simulink model "create_obs"  (R2019a)
settings: Solver=FixedStepAuto  StartTime=0.0  StopTime=100  FixedStep=1/4000  RelTol=1e-3
settings Model: Creator=brandlju  LastModifiedBy=brandlju
settings OptimizationCC: LocalBlockOutputs=off
settings RTWCC: SystemTargetFile=TwinCAT.tlc  GenCodeOnly=on  MakeCommand=make_tct  TemplateMakefile=tct_msbuild.tmf  Description=TwinCAT Target  GenerateReport=on  TargetLang=C++
settings STFCustomTargetCC: TargetLangStandard=C++03 (ISO)  CompOptLevelCompliant=on  MATLABClassNameForMDSCustomization=Simulink.SoftwareTarget.TargetSpecificTriggerConfigurationBase  SystemTargetFile=TwinCAT.tlc

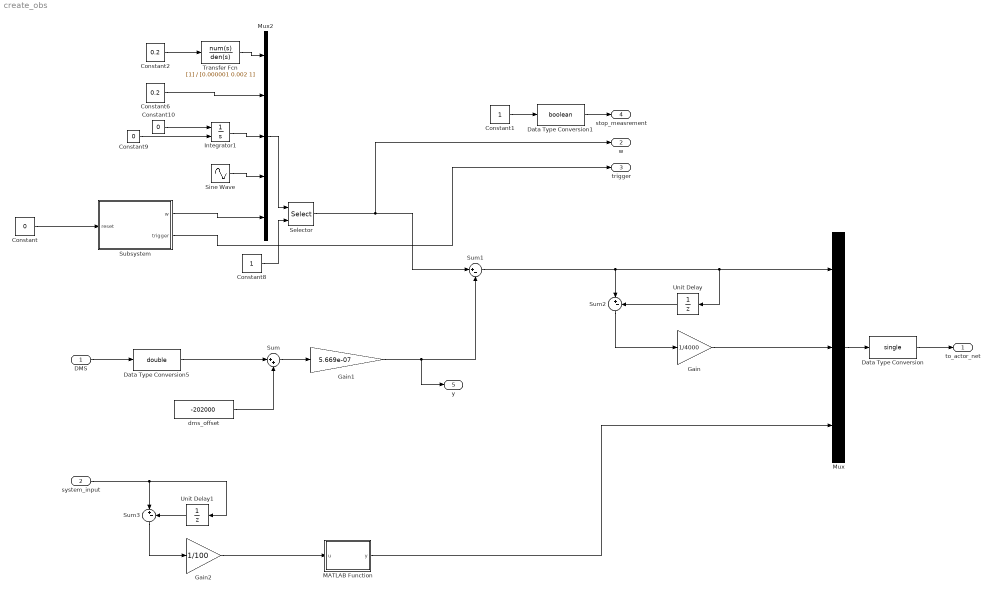
== system create_obs ==
  DMS : Inport  OutDataTypeStr=int32
  system_input : Inport  Port=2
  Constant : Constant  Value=0
  Constant1 : Constant
  Constant10 : Constant  Value=0
  Constant2 : Constant  Value=0.2
  Constant6 : Constant  Value=0.2
  Constant8 : Constant
  Constant9 : Constant  Value=0
  Data Type Conversion : DataTypeConversion  OutDataTypeStr=single
  Data Type Conversion1 : DataTypeConversion  OutDataTypeStr=boolean
  Data Type Conversion5 : DataTypeConversion  OutDataTypeStr=double
  Gain : Gain  Gain=1/4000
  Gain1 : Gain  Gain=5.669e-07
  Gain2 : Gain  Gain=1/100
  Integrator1 : Integrator  ExternalReset=either
  MATLAB Function : MATLAB Function  TreatAsAtomicUnit=on
  Mux : Mux  Inputs=3
  Mux2 : Mux  Inputs=5
  Selector : Selector  InputPortWidth=5  IndexOptions=Index vector (port)  Indices=[1 3]  OutputSizes=1
  Sine Wave : Sin  Amplitude=0.5  Bias=0.5  Frequency=0.1  SampleTime=0
  Subsystem : Subsystem
  Sum : Sum  Inputs=|++
  Sum1 : Sum  Inputs=|+-
  Sum2 : Sum  Inputs=|+-
  Sum3 : Sum  Inputs=|+-
  Transfer Fcn : TransferFcn  Denominator=[0.000001 0.002 1]
  Unit Delay : UnitDelay  SampleTime=-1  HasFrameUpgradeWarning=on
  Unit Delay1 : UnitDelay  SampleTime=-1  HasFrameUpgradeWarning=on
  "dms_offset " : Constant  Value=-202000
  to_actor_net : Outport  OutDataTypeStr=single
  w : Outport  Port=2
  trigger : Outport  Port=3
  stop_measrement : Outport  Port=4  OutDataTypeStr=boolean
  y : Outport  Port=5
  wires:
  "dms_offset "/1 -> Sum/2
  Data Type Conversion5/1 -> Sum/1
  Sum/1 -> Gain1/1
  DMS/1 -> Data Type Conversion5/1
  Gain1/1 -> y/1, Sum1/2
  Selector/1 -> w/1, Sum1/1
  Sum1/1 -> Sum2/1, Unit Delay/1, Mux/1
  Unit Delay/1 -> Sum2/2
  Gain/1 -> Mux/2
  Sum2/1 -> Gain/1
  Gain2/1 -> MATLAB Function/1(u)
  Sum3/1 -> Gain2/1
  system_input/1 -> Sum3/1, Unit Delay1/1
  Unit Delay1/1 -> Sum3/2
  MATLAB Function/1(y) -> Mux/3
  Mux/1 -> Data Type Conversion/1
  Data Type Conversion/1 -> to_actor_net/1
  Constant6/1 -> Mux2/2
  Sine Wave/1 -> Mux2/4
  Constant9/1 -> Integrator1/2
  Constant10/1 -> Integrator1/1
  Constant8/1 -> Selector/2
  Integrator1/1 -> Mux2/3
  Mux2/1 -> Selector/1
  Constant2/1 -> Transfer Fcn/1
  Transfer Fcn/1 -> Mux2/1
  Subsystem/1(w) -> Mux2/5
  Constant/1 -> Subsystem/1(reset)
  Data Type Conversion1/1 -> stop_measrement/1
  Constant1/1 -> Data Type Conversion1/1
  Subsystem/2(trigger) -> trigger/1

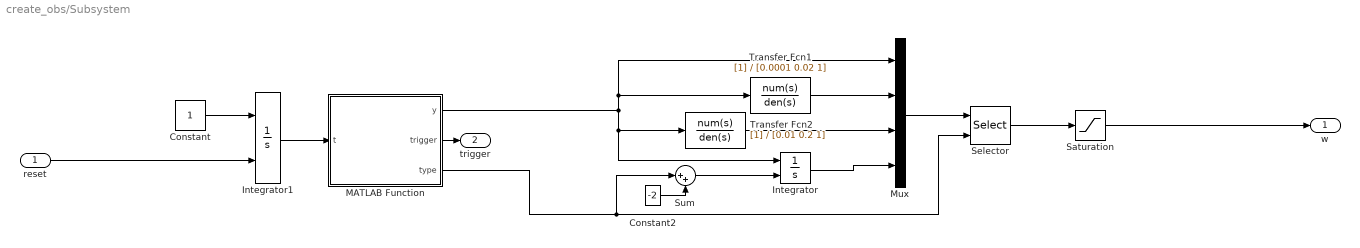
== system create_obs/Subsystem ==
  reset : Inport
  Constant : Constant
  Constant2 : Constant  Value=-2
  Integrator : Integrator  ExternalReset=rising
  Integrator1 : Integrator  ExternalReset=either
  MATLAB Function : MATLAB Function  TreatAsAtomicUnit=on
  Mux : Mux
  Saturation : Saturate  UpperLimit=1  LowerLimit=0.1
  Selector : Selector  IndexMode=Zero-based  InputPortWidth=4  IndexOptions=Index vector (port)  Indices=[1 3]  OutputSizes=1
  Sum : Sum  Inputs=|++
  Transfer Fcn1 : TransferFcn  Denominator=[0.0001 0.02 1]
  Transfer Fcn2 : TransferFcn  Denominator=[0.01 0.2 1]
  w : Outport
  trigger : Outport  Port=2
  wires:
  MATLAB Function/3(type) -> Sum/1, Selector/2
  MATLAB Function/1(y) -> Transfer Fcn1/1, Mux/1, Integrator/1, Transfer Fcn2/1
  Sum/1 -> Integrator/2
  Transfer Fcn2/1 -> Mux/3
  Integrator/1 -> Mux/4
  Mux/1 -> Selector/1
  Constant2/1 -> Sum/2
  Selector/1 -> Saturation/1
  Transfer Fcn1/1 -> Mux/2
  Constant/1 -> Integrator1/1
  Integrator1/1 -> MATLAB Function/1(t)
  reset/1 -> Integrator1/2
  MATLAB Function/2(trigger) -> trigger/1
  Saturation/1 -> w/1

== matlab function create_obs/Subsystem/MATLAB Function ==
  data: t input; y output; trigger output; type output
function [y, trigger, type] = fcn(t)
y = 0;
type = 0;
%% set trigger
if t > 1
    trigger = 1;
else
    trigger = 0;
end

%% steps
if t < 3
    y = 0.1;
    type = 0;
    return
elseif t < 5
    y = 0.11;
    type = 0;
    return
elseif t < 7
    y = 0.115;
    type = 0;
return
elseif t < 9
    y = 0.3;
    type = 0;
return
elseif t < 11
    y = 0.9;
    type = 0;
return
elseif t < 13
    y = 0.95;
    type = 0;
elseif t < 15
    y = 0.96;
    type = 0;
return
elseif t < 17
    y = 0.965;
    type = 0;
return
elseif t < 19
    y = 0.1;
    type = 0;
return


%% pt2 fast
elseif t < 24
    y = 0.1;
    type = 1;
    return
elseif t < 26
    y = 0.11;
    type = 1;
    return
elseif t < 28
    y = 0.115;
    type = 1;
return
elseif t < 30
    y = 0.3;
    type = 1;
return
elseif t < 32
    y = 0.9;
    type = 1;
return
elseif t < 34
    y = 0.95;
    type = 1;
elseif t < 36
    y = 0.96;
    type = 1;
return
elseif t < 38
    y = 0.965;
    type = 1;
return
elseif t < 40
    y = 0.1;
    type = 1;
return

%% pt2 slow
elseif t < 45
    y = 0.1;
    type = 2;
    return
elseif t < 47
    y = 0.11;
    type = 2;
    return
elseif t < 49
    y = 0.115;
    type = 2;
return
elseif t < 51
    y = 0.3;
    type = 2;
return
elseif t < 53
    y = 0.9;
    type = 2;
return
elseif t < 55
    y = 0.95;
    type = 2;
elseif t < 57
    y = 0.96;
    type = 2;
return
elseif t < 59
    y = 0.965;
    type = 2;
return
elseif t < 61
    y = 0.1;
    type = 2;
return

%% ramps
elseif t < 65
    y = 0.0;
    type = 3;
    return
elseif t < 66
    y = 0.0;
    type = 3;
    return
elseif t < 67
    y = +0.1;
    type = 3;
    return
elseif t < 68
    y = 0.0;
    type = 3;
    return
elseif t < 69
    y = +0.2;
    type = 3;
return
elseif t < 70
    y = 0.0;
    type = 3;
    return
elseif t < 71
    y = +0.01;
    type = 3;
return
elseif t < 72
    y = 0.0;
    type = 3;
    return
elseif t < 73
    y = 0.6;
    type = 3;
return
elseif t < 74
    y = 0.0;
    type = 3;
    return
elseif t < 75
    y = 0.0;
    type = 3;
elseif t < 77
    y = +0.001;
    type = 3;
return
elseif t < 76
    y = 0.0;
    type = 3;
    return
elseif t < 77
    y = -0.8;
    type = 3;
return
elseif t < 78
    y = -0.8;
    type = 3;
    return
elseif t < 79
    y = 0.0;
    type = 3;
return



end

end

== matlab function create_obs/MATLAB Function ==
  settings: updateMethod=DISCRETE
  data: u input; y output
function y = fcn(u)
persistent out
if isempty(out)
   out = u; 
end
if u ~= 0
   out = u; 
end

y = out;
